simulink model "Verifica_EIG_06072026"  (R2025b)
settings: Solver=VariableStepAuto  StartTime=0.0  StopTime=10.0  RelTol=1e-3
undefined symbols (not defined in the file): K_eig, u_bar, x0_sylv
settings Model: Creator=salvo  LastModifiedBy=salvo

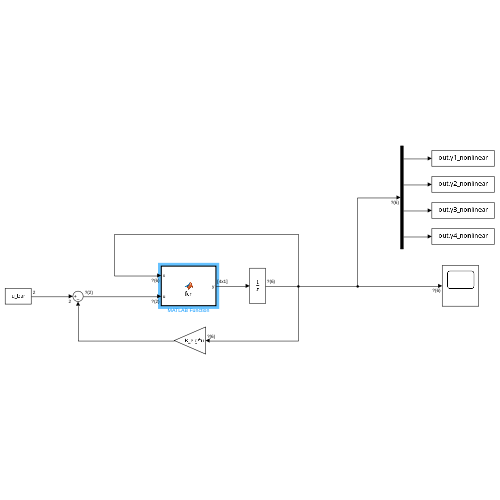
[thumbnail: Simulink's stored preview of the top-level diagram]
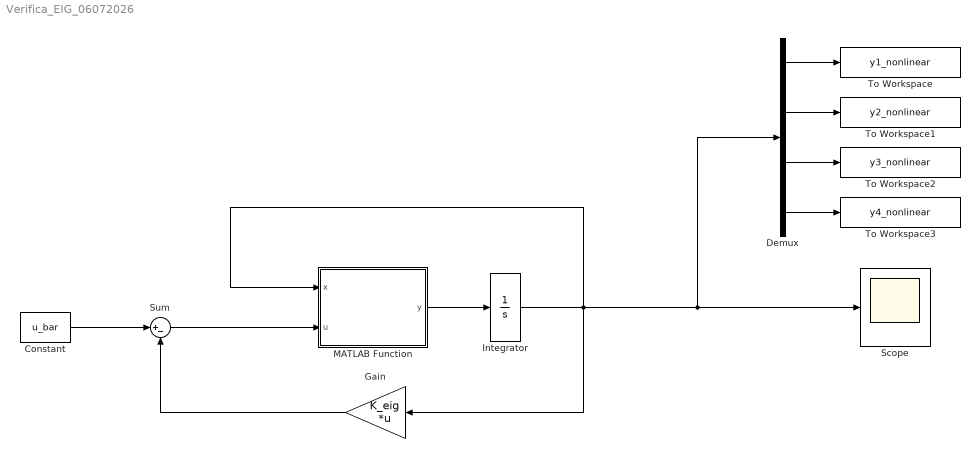
== system Verifica_EIG_06072026 ==
  Constant : Constant  Value=u_bar
  Demux : Demux
  Gain : Gain  Gain=K_eig  Multiplication=Matrix(K*u)
  Integrator : Integrator  InitialCondition=x0_sylv
  MATLAB Function : MATLAB Function  TreatAsAtomicUnit=on
  Scope : Scope
      settings: ActiveDisplayYMinimum=-0.13215665313460279  ActiveDisplayYMaximum=0.18940987821142502
  Sum : Sum  Inputs=|+-
  To Workspace : ToWorkspace  VariableName=y1_nonlinear  SaveFormat=Timeseries  SampleTime=-1
  To Workspace1 : ToWorkspace  VariableName=y2_nonlinear  SaveFormat=Timeseries  SampleTime=-1
  To Workspace2 : ToWorkspace  VariableName=y3_nonlinear  SaveFormat=Timeseries  SampleTime=-1
  To Workspace3 : ToWorkspace  VariableName=y4_nonlinear  SaveFormat=Timeseries  SampleTime=-1
  wires:
  MATLAB Function/1(y) -> Integrator/1
  Integrator/1 -> Gain/1, Demux/1, Scope/1, MATLAB Function/1(x)
  Constant/1 -> Sum/1
  Sum/1 -> MATLAB Function/2(u)
  Gain/1 -> Sum/2
  Demux/1 -> To Workspace/1
  Demux/2 -> To Workspace1/1
  Demux/3 -> To Workspace2/1
  Demux/4 -> To Workspace3/1

== matlab function Verifica_EIG_06072026/MATLAB Function ==
  data: x input; u input; y output
function y = fcn(x, u)

m = 1.5;
J = 0.025;
g = 9.81;

px = x(1);
pz = x(2);
theta = x(3);
dpx = x(4);
dpz = x(5);
dtheta = x(6);
    
T = u(1);
tau = u(2);
    
ddpx = -(T/m)*sin(theta);
ddpz = (T/m)*cos(theta) - g;
ddtheta = tau/J;
    
y = [dpx;
     dpz;
     dtheta;
     ddpx;
     ddpz;
     ddtheta];
